simulink subsystem "Light_Sensor_Simulation_ThorneFleissner"  (R2020b)
settings: Solver=VariableStepAuto  StartTime=0.0  StopTime=10.0  RelTol=1e-3
values from neighbouring files (symbols this model uses):
  Map = im2double(Map).*255    [Configuration.m]    (also in ConfigurationCreation.m)
settings Model: Creator=rthom  LastModifiedBy=dffleiss

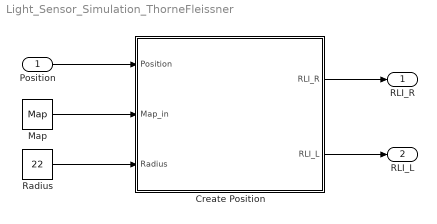
== system Light_Sensor_Simulation_ThorneFleissner ==
  Position : Inport
  Create Position : MATLAB Function  TreatAsAtomicUnit=on
  Map : Constant  Value=Map
  Radius : Constant  Value=22
  RLI_R : Outport
  RLI_L : Outport  Port=2
  wires:
  Create Position/2(RLI_L) -> RLI_L/1
  Create Position/1(RLI_R) -> RLI_R/1
  Position/1 -> Create Position/1(Position)
  Map/1 -> Create Position/2(Map_in)
  Radius/1 -> Create Position/3(Radius)

== matlab function Light_Sensor_Simulation_ThorneFleissner/Create Position ==
  settings: updateMethod=DISCRETE
  data: Position input; Map_in input; Radius input; RLI_R output; RLI_L output
function [RLI_R,RLI_L] = CreatePosition(Position, Map_in, Radius)
persistent Map
if isempty(Map)
    Map = Map_in;
end

%Position of Light Sensors (based on EV Center of Mass)
    x = Position(1) + 0.6*cos(Position(3));%Calculate x position of front of vehicle
    y = Position(2) + 0.6*sin(Position(3));%Calculate y position of front of vehicle

    %Need to change so that bottom left is 0,0. Need to find what top value
    %is in m and pixels.
    TopOptiTrack = 2.936;%m, top boundary of map from OptiTrack
    LeftOptiTrack = -1.9;%m, left boundary of map from OptiTrack

    TopPixel = 69;%pixel, top boundary of map from image
    LeftPixel = 71;%pixel, left boundary of map from image

    xScale = 144.4175;%Scale factor between pixels and real values from OptiTrack for x
    yScale = -140.7979;%Scale factor between pixels and real values from OptiTrack for y

    x_Pixel = LeftPixel + (xScale*(x - LeftOptiTrack));%Convert the x position of front of vehicle into pixels
    y_Pixel = TopPixel + (yScale*(y - TopOptiTrack));%Convert the y position of front of vehicle into pixels


    x_LeftSensor = x_Pixel - 34*sin(Position(3));%Calculate Left Sensor x Position in pixels
    y_LeftSensor = y_Pixel - 34*cos(Position(3));%Calculate Left Sensor y Position in pixels

    x_RightSensor = x_Pixel + 34*sin(Position(3));%Calculate Right Sensor x Position in pixels
    y_RightSensor = y_Pixel + 34*cos(Position(3));%Calculate Right Sensor y Position in pixels
%RLI Shared Code
    X = -Radius:Radius;%Define size of circle in x direction
    Y = -Radius:Radius;%Define size of circle in y direction
    [MX,MY] = meshgrid(X,Y);%Create meshgrid (square) the size of the radius
    
    Circle = MX.^2 + MY.^2 <= Radius^2;%Create mask in shape of circle using meshgrid values
%Right RLI
    X_Boundary_R = round(x_RightSensor - Radius:x_RightSensor + Radius);%Calculate x coordinate boundary of the light sensor
    Y_Boundary_R = round(y_RightSensor - Radius:y_RightSensor + Radius);%Calculate y coordinate boundary of the light sensor

    Area_R = Map(Y_Boundary_R, X_Boundary_R);%Define area within the map. Indexing is Map(y,x)
    
    RLI_R = sum(Area_R.*Circle,'all') / sum(Circle,'all');%Calculate the average of values over the circular area;
%     RLI_R = round(RLI_R*.7 + 10);%I don't know what this is for yet. 

%Left RLI
    X_Boundary_L = round(x_LeftSensor - Radius:x_LeftSensor + Radius);%Calculate x coordinate boundary of the light sensor
    Y_Boundary_L = round(y_LeftSensor - Radius:y_LeftSensor + Radius);%Calculate y coordinate boundary of the light sensor

    Area_L = Map(Y_Boundary_L, X_Boundary_L);%Define area within the map. Indexing is Map(y,x)
    
    RLI_L = sum(Area_L.*Circle,'all') / sum(Circle,'all');%Calculate the average of values over the circular area;
%     RLI_L = round(RLI_L*.7 + 10);%I don't know what this is for yet.
end
